simulink model "dc_motor_ann"  (R2024a)
settings: Solver=VariableStepAuto  StartTime=0.0  StopTime=10.0  RelTol=1e-3
libraries: simulink x1
settings Model: Creator=Aman  LastModifiedBy=Aman

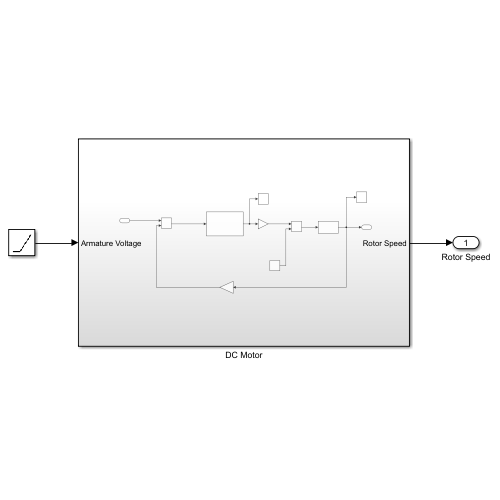
[thumbnail: Simulink's stored preview of the top-level diagram]
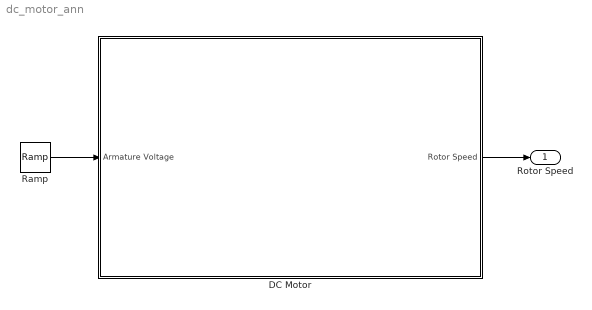
== system dc_motor_ann ==
  DC Motor : Subsystem
  Ramp : simulink/Sources/Ramp  slope=0.5  start=0  InitialOutput=0
  Rotor Speed : Outport
  wires:
  DC Motor/1(Rotor Speed) -> Rotor Speed/1
  Ramp/1 -> DC Motor/1(Armature Voltage)

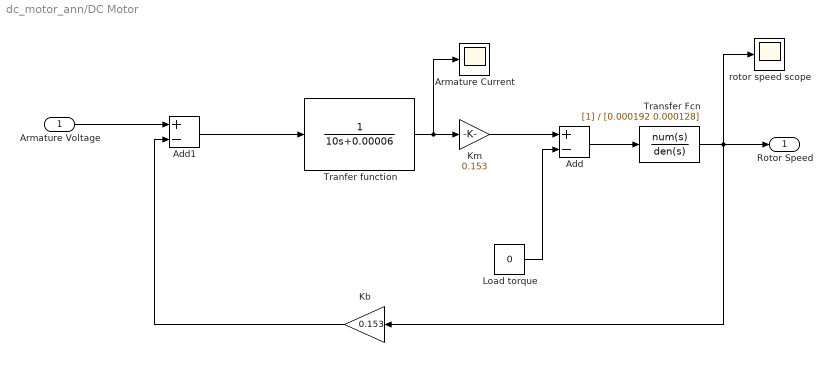
== system dc_motor_ann/DC Motor ==
  Armature Voltage : Inport
  Add : Sum  Inputs=+-
  Add1 : Sum  Inputs=+-
  Armature Current : Scope
  Kb : Gain  Gain=0.153
  Km : Gain  Gain=0.153
  Load torque : Constant  Value=0
  Tranfer function : TransferFcn  Denominator=[10 0.00006]
  Transfer Fcn : TransferFcn  Denominator=[0.000192 0.000128]
  rotor speed scope : Scope
  Rotor Speed : Outport
  wires:
  Km/1 -> Add/1
  Add1/1 -> Tranfer function/1
  Tranfer function/1 -> Armature Current/1, Km/1
  Transfer Fcn/1 -> Rotor Speed/1, rotor speed scope/1, Kb/1
  Load torque/1 -> Add/2
  Add/1 -> Transfer Fcn/1
  Kb/1 -> Add1/2
  Armature Voltage/1 -> Add1/1
